simulink model "YY"  (R2018a)
settings: Solver=VariableStepAuto  StartTime=0.0  StopTime=0.2  RelTol=1e-3
libraries: powerlib x10, peRmsMeasurement x8
settings Model: Creator=ROY D. DEBOPRIYA  LastModifiedBy=ROY D. DEBOPRIYA

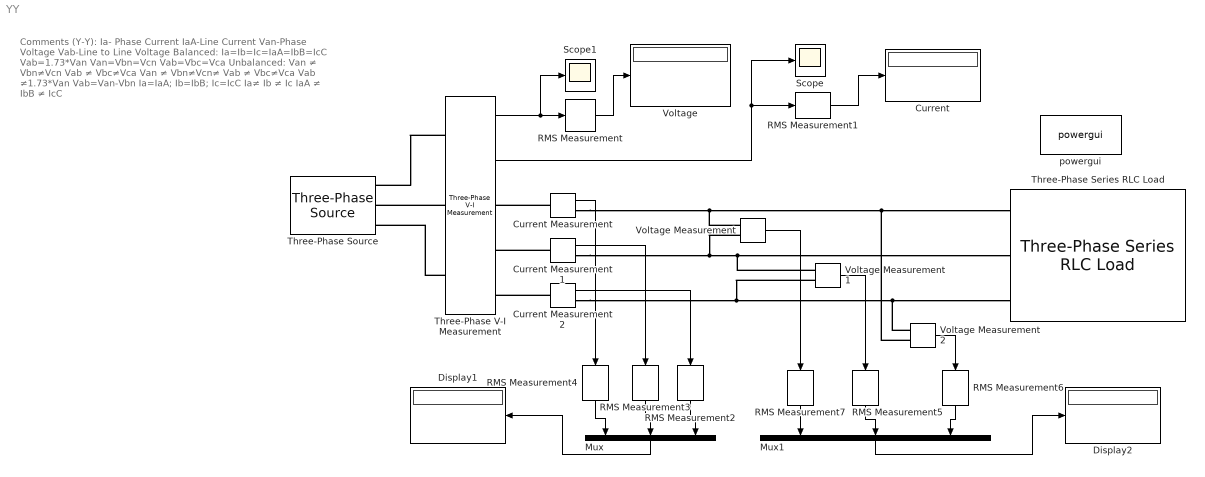
== system YY ==
  note: Comments (Y-Y):
      | Ia- Phase Current
      | IaA-Line Current
      | Van-Phase Voltage
      | Vab-Line to Line Voltage
      | Balanced:
      | Ia=Ib=Ic=IaA=IbB=IcC
      | Vab=1.73*Van
      | Van=Vbn=Vcn
      | Vab=Vbc=Vca
      | Unbalanced:
      | Van ≠ Vbn≠Vcn
      | Vab ≠ Vbc≠Vca
      | Van ≠ Vbn≠Vcn≠ Vab ≠ Vbc≠Vca
      | Vab ≠1.73*Van
      | Vab=Van-Vbn
      | Ia=IaA; Ib=IbB; Ic=IcC
      | Ia≠ Ib ≠ Ic
      | IaA ≠ IbB ≠ IcC
  Current : Display
  Current Measurement : powerlib/Measurements/Current Measurement  PhasorSimulation=off  OutputType=Complex  PSBequivalent=0
  Current Measurement1 : powerlib/Measurements/Current Measurement  PhasorSimulation=off  OutputType=Complex  PSBequivalent=0
  Current Measurement2 : powerlib/Measurements/Current Measurement  PhasorSimulation=off  OutputType=Complex  PSBequivalent=0
  Display1 : Display
  Display2 : Display
  Mux : Mux  Inputs=3
  Mux1 : Mux  Inputs=3
  RMS Measurement{,1..7} (8 alike) : peRmsMeasurement/RMS Measurement  OverrideUsingVariant=Total  F=60  SpecifyHarmonics=off  K=[0 1 2]  Ts=0
  Scope : Scope
  Scope1 : Scope
  Three-Phase Series RLC Load : powerlib/Elements/Three-Phase Series RLC Load  LConnTagsString=A|B|C  Configuration=Y (grounded)  NominalVoltage=1000  Vabc=[230 230 230]  Vabcp=[1e3 1e3 1e3]  NominalFrequency=50  UnbalancedPower=on  ActivePower=10e3  InductivePower=100  CapacitivePower=100  Pabc=[1000 1000 1000]  QLabc=[0 0 0]  QCabc=[0 0 0]  Pabcp=[10e3 9e3 11e3]  QLabcp=[100 90 110]  QCabcp=[100 90 110]  Measurements=None  LoadType=constant Z
  Three-Phase V-I Measurement : powerlib/Measurements/Three-Phase V-I Measurement  VoltageMeasurement=phase-to-ground  SetLabelV=off  LabelV=Vabc  Vpu=off  VpuLL=off  CurrentMeasurement=yes  SetLabelI=off  LabelI=Iabc  Ipu=off  Pbase=100e6  Vbase=500e3  OutputType=Complex  PhasorSimulation=off  PSBequivalent=0
  Three-Phase Source : powerlib/Electrical Sources/Three-Phase Source  InternalConnection=Yn  VoltagePhases=off  Voltage=25e3  PhaseAngle=0  Voltage_phases=[25e3 25e3 25e3]/sqrt(3)  PhaseAngles_phases=[0 -120 +120]  Frequency=60  NonIdealSource=on  SpecifyImpedance=off  Resistance=0.8929  Inductance=16.58e-3  ShortCircuitLevel=100e6  BaseVoltage=25e3  XRratio=7  BusType=swing  Pref=10e3  Qref=0  Prefabc=[10e3, 10e3, 10e3]  Qrefabc=[0, 0, 0]  Qmin=-inf  Qmax=inf
  Voltage : Display
  Voltage Measurement : powerlib/Measurements/Voltage Measurement  PhasorSimulation=off  OutputType=Complex  PSBequivalent=0
  Voltage Measurement1 : powerlib/Measurements/Voltage Measurement  PhasorSimulation=off  OutputType=Complex  PSBequivalent=0
  Voltage Measurement2 : powerlib/Measurements/Voltage Measurement  PhasorSimulation=off  OutputType=Complex  PSBequivalent=0
  powergui : powerlib/powergui  Priority=1  SimulationMode=Continuous  SampleTime=50e-6  frequency=60  Iterations=50  frequencyindice=60  Pbase=100e6  ErrMax=1e-4  UnitsV=kV  UnitsW=MW  buscounter=0  FunctionMessages=off  echomessages=off  EnableUseOfTLC=off  CurrentSourceSwitches=off  DisableSnubberDevices=off  DisableRonSwitches=off  DisableVfSwitches=off  DisplayEquations=off  SolverType=Tustin/Backward Euler (TBE)  Interpol=off  ExternalGateDelay=off  methode=off  Ts=100  x0status=blocks  SPID=on  SwTol=0  HookPort=off  RestoreLinks=warning  ResistiveCurrentMeasurement=off  Frange=[0:2:500]  Ylog=off  Xlog=on  ShowGrid=off  save=off  variable=ZData  structure=0  ZoomFFT=off  StartTime=0.0  cycles=1  DisplayStyle=1  fundamental=60  FreqAxis=off  MaxFrequency=1000  frequencyindicesteady=1  RmsSteady=1  display=off
  wires:
  Three-Phase V-I Measurement/2 -> RMS Measurement1/1, Scope/1
  RMS Measurement1/1 -> Current/1
  Three-Phase V-I Measurement/1 -> Scope1/1, RMS Measurement/1
  Current Measurement/1 -> RMS Measurement4/1
  Current Measurement1/1 -> RMS Measurement3/1
  Current Measurement2/1 -> RMS Measurement2/1
  RMS Measurement4/1 -> Mux/1
  RMS Measurement3/1 -> Mux/2
  RMS Measurement2/1 -> Mux/3
  Mux/1 -> Display1/1
  Voltage Measurement/1 -> RMS Measurement7/1
  Voltage Measurement1/1 -> RMS Measurement5/1
  Voltage Measurement2/1 -> RMS Measurement6/1
  RMS Measurement7/1 -> Mux1/1
  RMS Measurement5/1 -> Mux1/2
  RMS Measurement6/1 -> Mux1/3
  Mux1/1 -> Display2/1
  RMS Measurement/1 -> Voltage/1
  connections:
  Three-Phase V-I Measurement/LConn1 -- Three-Phase Source/RConn1
  Three-Phase V-I Measurement/LConn2 -- Three-Phase Source/RConn2
  Three-Phase V-I Measurement/LConn3 -- Three-Phase Source/RConn3
  Current Measurement/RConn1 -- Three-Phase Series RLC Load/LConn1 -- Voltage Measurement2/LConn2 -- Voltage Measurement/LConn1
  Current Measurement/LConn1 -- Three-Phase V-I Measurement/RConn1
  Current Measurement1/LConn1 -- Three-Phase V-I Measurement/RConn2
  Current Measurement1/RConn1 -- Voltage Measurement1/LConn1 -- Three-Phase Series RLC Load/LConn2 -- Voltage Measurement/LConn2
  Current Measurement2/LConn1 -- Three-Phase V-I Measurement/RConn3
  Current Measurement2/RConn1 -- Voltage Measurement1/LConn2 -- Three-Phase Series RLC Load/LConn3 -- Voltage Measurement2/LConn1
